simulink model "ZeroCrossDetection_UsingEnabledSubsystem"  (R2024b)
settings: Solver=VariableStepAuto  StartTime=0.0  StopTime=10.0  MaxStep=1e-4  RelTol=1e-3
libraries: simulink x1
settings Model: Creator=MOHAMED  LastModifiedBy=MOHAMED

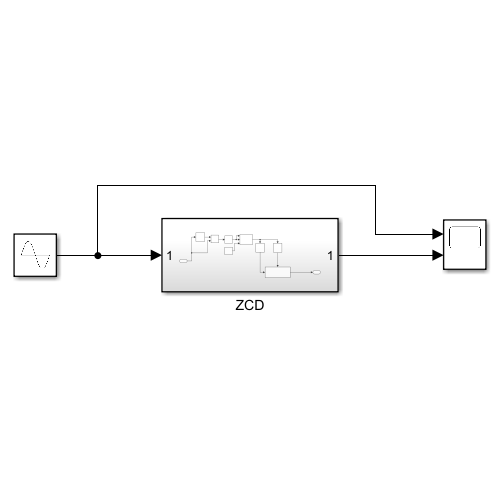
[thumbnail: Simulink's stored preview of the top-level diagram]
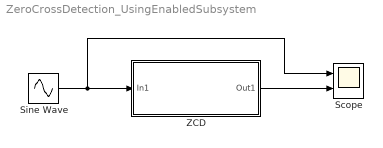
== system ZeroCrossDetection_UsingEnabledSubsystem ==
  Scope : Scope  NumInputPorts=2
  Sine Wave : Sin  Amplitude=5  Frequency=2*pi/(2.5)  SampleTime=0
  ZCD : Subsystem
  wires:
  Sine Wave/1 -> Scope/1, ZCD/1(In1)
  ZCD/1(Out1) -> Scope/2

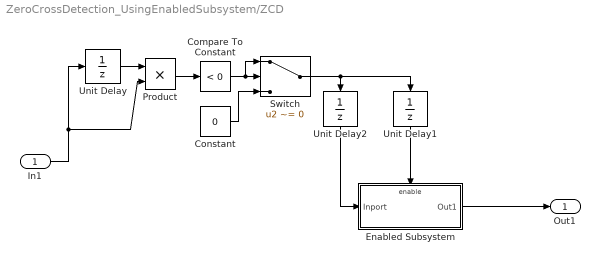
== system ZeroCrossDetection_UsingEnabledSubsystem/ZCD ==
  In1 : Inport
  Compare To Constant : simulink/Logic and Bit Operations/Compare To Constant  relop=<  const=0  OutDataTypeStr=boolean
  Constant : Constant  Value=0
  Enabled Subsystem : Subsystem  TreatAsAtomicUnit=on
  Product : Product
  Switch : Switch  Criteria=u2 ~= 0  SaturateOnIntegerOverflow=off  InputSameDT=off
  Unit Delay : UnitDelay  SampleTime=1e-3  HasFrameUpgradeWarning=on
  Unit Delay1 : UnitDelay  SampleTime=1e-3  HasFrameUpgradeWarning=on
  Unit Delay2 : UnitDelay  SampleTime=1e-3/2  HasFrameUpgradeWarning=on
  Out1 : Outport
  wires:
  Constant/1 -> Switch/3
  Compare To Constant/1 -> Switch/1, Switch/2
  Unit Delay1/1 -> Enabled Subsystem/Enable
  Switch/1 -> Unit Delay2/1, Unit Delay1/1
  Unit Delay2/1 -> Enabled Subsystem/1(Inport)
  In1/1 -> Product/2, Unit Delay/1
  Product/1 -> Compare To Constant/1
  Unit Delay/1 -> Product/1
  Enabled Subsystem/1(Out1) -> Out1/1

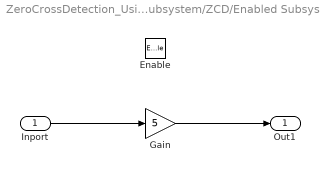
== system ZeroCrossDetection_UsingEnabledSubsystem/ZCD/Enabled Subsystem ==
  Inport : Inport
  Enable : EnablePort  StatesWhenEnabling=reset
  Gain : Gain  Gain=5
  Out1 : Outport
  wires:
  Gain/1 -> Out1/1
  Inport/1 -> Gain/1
